simulink model "Q3_model"  (R2020b)
settings: Solver=VariableStepAuto  StartTime=0.0  StopTime=10.0  RelTol=1e-3
values from neighbouring files (symbols this model uses):
  a = 0.5    [Q3.m]    (also in matlab.mat)
  Lss = 80    [Q3.m]    (also in matlab.mat)
  M = 20    [Q3.m]    (also in matlab.mat)
  Vss = 100    [Q3.m]    (also in matlab.mat)
  w_ss = x_ss(1)    [Q3.m]    (also in matlab.mat = 0.0387596899225)
  z_ss = x_ss(2)    [Q3.m]    (also in matlab.mat = 0.100775193798)
  zf = 0.1    [Q3.m]    (also in matlab.mat)
settings Model: Creator=HP  LastModifiedBy=HP

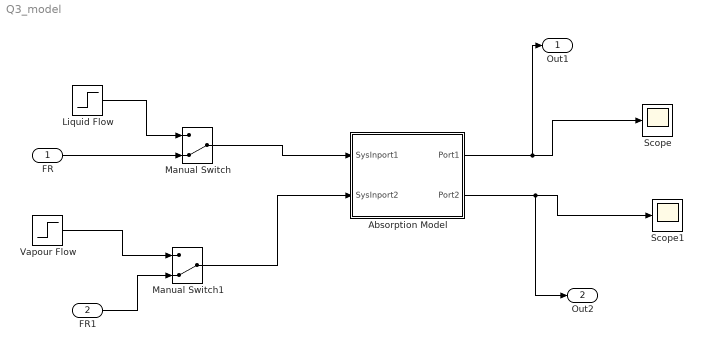
== system Q3_model ==
  FR : Inport
  FR1 : Inport  Port=2
  Absorption Model : Subsystem  mask(Differential Equation Editor (DEE)){}
      settings: OpenFcn=diffeqed
      mask Display: disp('abs')
  Liquid Flow : Step  Time=0  Before=Lss  After=Lss*1.05  SampleTime=0
  Manual Switch : ManualSwitch  CurrentSetting=0
  Manual Switch1 : ManualSwitch  CurrentSetting=0
  Scope : Scope
  Scope1 : Scope
  Vapour Flow : Step  Time=0  Before=Vss  After=Vss  SampleTime=0
  Out1 : Outport
  Out2 : Outport  Port=2
  wires:
  Absorption Model/1(Port1) -> Out1/1, Scope/1
  Absorption Model/2(Port2) -> Out2/1, Scope1/1
  Liquid Flow/1 -> Manual Switch/1
  FR/1 -> Manual Switch/2
  Vapour Flow/1 -> Manual Switch1/1
  FR1/1 -> Manual Switch1/2
  Manual Switch1/1 -> Absorption Model/2(SysInport2)
  Manual Switch/1 -> Absorption Model/1(SysInport1)

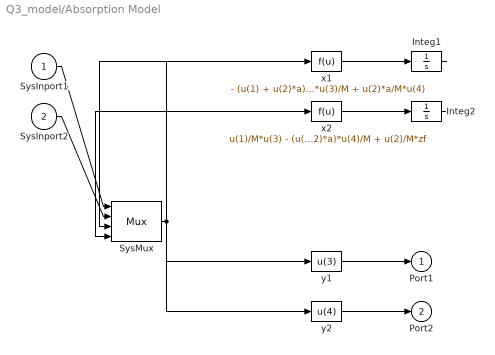
== system Q3_model/Absorption Model ==
  SysInport1 : Inport
  SysInport2 : Inport  Port=2
  Integ1 : Integrator  InitialCondition=w_ss
  Integ2 : Integrator  InitialCondition=z_ss
  SysMux : Mux
  x1 : Fcn  Expr=- (u(1) + u(2)*a)*u(3)/M + u(2)*a/M*u(4)
  x2 : Fcn  Expr=u(1)/M*u(3) - (u(1) + u(2)*a)*u(4)/M + u(2)/M*zf
  y1 : Fcn  Expr=u(3)
  y2 : Fcn  Expr=u(4)
  Port1 : Outport  InitialOutput=0
  Port2 : Outport  Port=2
  wires:
  SysInport1/1 -> SysMux/1
  SysInport2/1 -> SysMux/2
  SysMux/1 -> x1/1, x2/1, y1/1, y2/1
  x1/1 -> Integ1/1
  Integ1/1 -> SysMux/3
  x2/1 -> Integ2/1
  Integ2/1 -> SysMux/4
  y1/1 -> Port1/1
  y2/1 -> Port2/1
